simulink model "final"  (R2025b)
settings: Solver=FixedStepAuto  StartTime=0.0  StopTime=20.0  FixedStep=0.001  RelTol=1e-3
values from neighbouring files (symbols this model uses):
  c_d = 0.05    [final_param.m]
  Dm = 1e-3    (= 0.001)    [final_param.m]
  Jm = 0.1e-3    (= 0.0001)    [final_param.m]
  k_s = 0.2    [final_param.m]
  L = [L11]    [final_param.m]
  Ld = 0.01    [final_param.m]
  Lq = 0.02    [final_param.m]
  p = 2    [final_param.m]
  Phi = 0.1    [final_param.m]
  Rs = 0.38    [final_param.m]
libraries: fl_lib x50, nesl_utility x50, ee_lib x15, eeTransforms x10, simulink x1
(part 3 of 3)

== system final/Subsystem5/Plant/MechSensor ==
  Ideal Rotational Motion Sensor : fl_lib/Mechanical/Mechanical Sensors/Ideal Rotational Motion Sensor  reference=foundation.enum.MeasurementReference.difference  acceleration_port=false  velocity_port=true  position_port=true  wrap_angle=simscape.enum.onoff.off  offset=0 rad
  Ideal Torque Sensor : fl_lib/Mechanical/Mechanical Sensors/Ideal Torque Sensor
  PS-Simulink Converter : nesl_utility/PS-Simulink Converter  PhysicalDomain=network_engine_domain  SubClassName=ps_output  LeftPortType=input  RightPortType=output  PseudoPeriodic=off  Frequencies=[]  VectorFormat=1-D array  Unit=1  AffineConversion=off
  PS-Simulink Converter1 : nesl_utility/PS-Simulink Converter  PhysicalDomain=network_engine_domain  SubClassName=ps_output  LeftPortType=input  RightPortType=output  PseudoPeriodic=off  Frequencies=[]  VectorFormat=1-D array  Unit=1  AffineConversion=off
  PS-Simulink Converter2 : nesl_utility/PS-Simulink Converter  PhysicalDomain=network_engine_domain  SubClassName=ps_output  LeftPortType=input  RightPortType=output  PseudoPeriodic=off  Frequencies=[]  VectorFormat=1-D array  Unit=1  AffineConversion=off
  R1 : PMIOPort  Side=Left
  C1 : PMIOPort  Port=2  Side=Left
  R2 : PMIOPort  Port=3  Side=Right
  C2 : PMIOPort  Port=4  Side=Right
  wm : Outport  VectorParamsAs1DForOutWhenUnconnected=off
  thm : Outport  Port=2  VectorParamsAs1DForOutWhenUnconnected=off
  Tm : Outport  Port=3  VectorParamsAs1DForOutWhenUnconnected=off
  wires:
  PS-Simulink Converter/1 -> thm/1
  PS-Simulink Converter1/1 -> Tm/1
  PS-Simulink Converter2/1 -> wm/1
  connections:
  Ideal Rotational Motion Sensor/RConn3 -- PS-Simulink Converter/LConn1
  Ideal Rotational Motion Sensor/RConn1 -- C2/RConn1 -- C1/RConn1
  Ideal Torque Sensor/LConn1 -- R1/RConn1
  Ideal Torque Sensor/RConn1 -- R2/RConn1 -- Ideal Rotational Motion Sensor/LConn1
  PS-Simulink Converter1/LConn1 -- Ideal Torque Sensor/RConn2
  Ideal Rotational Motion Sensor/RConn2 -- PS-Simulink Converter2/LConn1

== system final/Subsystem1/Controller2/DriverPeripherals/Break Algebraic Loop ==
  In1 : Inport
  Demux : Demux  Outputs=3
  Mux : Mux  Inputs=3
  Transfer Fcn : TransferFcn  Denominator=[1e-6 1]
  Transfer Fcn1 : TransferFcn  Denominator=[1e-6 1]
  Transfer Fcn2 : TransferFcn  Denominator=[1e-6 1]
  Out1 : Outport
  wires:
  In1/1 -> Demux/1
  Demux/1 -> Transfer Fcn/1
  Transfer Fcn/1 -> Mux/1
  Demux/2 -> Transfer Fcn1/1
  Transfer Fcn1/1 -> Mux/2
  Demux/3 -> Transfer Fcn2/1
  Transfer Fcn2/1 -> Mux/3
  Mux/1 -> Out1/1

== system final/Subsystem1/Controller2/FOC/CurrentController ==
  Iqref : Inport
  Id : Inport  Port=2
  Iq : Inport  Port=3
  we : Inport  Port=4
  Integrator : Integrator
  MATLAB Function : MATLAB Function  TreatAsAtomicUnit=on
  Scope : Scope
      settings: ActiveDisplayYMinimum=-0.021972241997855933  ActiveDisplayYMaximum=0.011100987286103392  DataLoggingVariableName=ScopeData15
  Vdref : Outport  VectorParamsAs1DForOutWhenUnconnected=off
  Vqref : Outport  Port=2  VectorParamsAs1DForOutWhenUnconnected=off
  wires:
  MATLAB Function/2(Vd) -> Vdref/1
  Iqref/1 -> MATLAB Function/2(i_q_ref)
  MATLAB Function/4(e_q_bar) -> Scope/1
  we/1 -> MATLAB Function/5(we)
  Id/1 -> MATLAB Function/4(i_d)
  Iq/1 -> MATLAB Function/3(i_q)
  Integrator/1 -> MATLAB Function/1(z_q)
  MATLAB Function/1(Vq) -> Vqref/1
  MATLAB Function/3(dz_q) -> Integrator/1

== system final/Subsystem1/Controller2/FOC/VelocityController ==
  wmref : Inport
  wm : Inport  Port=2
  Gain : Gain  Gain=1/(3/2*p*Phi)
  Integrator : Integrator
  Integrator1 : Integrator
  MATLAB Function : MATLAB Function  TreatAsAtomicUnit=on
  Iqref : Outport  VectorParamsAs1DForOutWhenUnconnected=off
  wires:
  MATLAB Function/2(dot_bar_w) -> Integrator/1
  wm/1 -> MATLAB Function/2(w_m)
  MATLAB Function/1(u_cmd) -> Gain/1
  Integrator/1 -> MATLAB Function/3(bar_w)
  Gain/1 -> Iqref/1
  wmref/1 -> MATLAB Function/1(w_ref)
  MATLAB Function/3(dot_xi) -> Integrator1/1
  Integrator1/1 -> MATLAB Function/4(xi)

== system final/Subsystem1/Controller2/FOC/abc2dq ==
  Iabc : Inport
  thetae : Inport  Port=2
  Demux1 : Demux  Outputs=3
  Park Transform : eeTransforms/Park Transform  AxisAlignment=D-axis  PowerInvariant=off
  Terminator : Terminator
  Id : Outport  VectorParamsAs1DForOutWhenUnconnected=off
  Iq : Outport  Port=2  VectorParamsAs1DForOutWhenUnconnected=off
  wires:
  Iabc/1 -> Park Transform/1
  thetae/1 -> Park Transform/2
  Demux1/3 -> Terminator/1
  Park Transform/1 -> Demux1/1
  Demux1/1 -> Id/1
  Demux1/2 -> Iq/1

== system final/Subsystem1/Controller2/FOC/dq2abc ==
  Vd : Inport
  Vq : Inport  Port=2
  thetae : Inport  Port=3
  Constant : Constant  Value=0
  Inverse Park Transform : eeTransforms/Inverse Park Transform  AxisAlignment=D-axis  PowerInvariant=off
  Mux : Mux  Inputs=3
  Vabc : Outport  VectorParamsAs1DForOutWhenUnconnected=off
  wires:
  thetae/1 -> Inverse Park Transform/2
  Constant/1 -> Mux/3
  Mux/1 -> Inverse Park Transform/1
  Vd/1 -> Mux/1
  Inverse Park Transform/1 -> Vabc/1
  Vq/1 -> Mux/2

== system final/Subsystem1/Controller2/FOC/thm2the ==
  thm : Inport
  Constant : Constant  Value=2*pi
  Mod : Math  Operator=mod  SignedPower=on
  PolePairs : Gain  Gain=p
  the : Outport  VectorParamsAs1DForOutWhenUnconnected=off
  wires:
  Constant/1 -> Mod/2
  PolePairs/1 -> Mod/1
  Mod/1 -> the/1
  thm/1 -> PolePairs/1

== system final/Subsystem1/Controller2/FOC/wm2we ==
  wm : Inport
  PolePairs : Gain  Gain=p
  we : Outport  VectorParamsAs1DForOutWhenUnconnected=off
  wires:
  wm/1 -> PolePairs/1
  PolePairs/1 -> we/1

== system final/Subsystem2/Controller2/DriverPeripherals/Break Algebraic Loop ==
  In1 : Inport
  Demux : Demux  Outputs=3
  Mux : Mux  Inputs=3
  Transfer Fcn : TransferFcn  Denominator=[1e-6 1]
  Transfer Fcn1 : TransferFcn  Denominator=[1e-6 1]
  Transfer Fcn2 : TransferFcn  Denominator=[1e-6 1]
  Out1 : Outport
  wires:
  In1/1 -> Demux/1
  Demux/1 -> Transfer Fcn/1
  Transfer Fcn/1 -> Mux/1
  Demux/2 -> Transfer Fcn1/1
  Transfer Fcn1/1 -> Mux/2
  Demux/3 -> Transfer Fcn2/1
  Transfer Fcn2/1 -> Mux/3
  Mux/1 -> Out1/1

== system final/Subsystem2/Controller2/FOC/CurrentController ==
  Iqref : Inport
  Id : Inport  Port=2
  Iq : Inport  Port=3
  we : Inport  Port=4
  Integrator : Integrator
  MATLAB Function : MATLAB Function  TreatAsAtomicUnit=on
  Scope : Scope
      settings: ActiveDisplayYMinimum=-0.021972241997855933  ActiveDisplayYMaximum=0.011100987286103392  DataLoggingVariableName=ScopeData15
  Vdref : Outport  VectorParamsAs1DForOutWhenUnconnected=off
  Vqref : Outport  Port=2  VectorParamsAs1DForOutWhenUnconnected=off
  wires:
  MATLAB Function/2(Vd) -> Vdref/1
  Iqref/1 -> MATLAB Function/2(i_q_ref)
  MATLAB Function/4(e_q_bar) -> Scope/1
  we/1 -> MATLAB Function/5(we)
  Id/1 -> MATLAB Function/4(i_d)
  Iq/1 -> MATLAB Function/3(i_q)
  Integrator/1 -> MATLAB Function/1(z_q)
  MATLAB Function/1(Vq) -> Vqref/1
  MATLAB Function/3(dz_q) -> Integrator/1

== system final/Subsystem2/Controller2/FOC/VelocityController ==
  wmref : Inport
  wm : Inport  Port=2
  Gain : Gain  Gain=1/(3/2*p*Phi)
  Integrator : Integrator
  Integrator1 : Integrator
  MATLAB Function : MATLAB Function  TreatAsAtomicUnit=on
  Iqref : Outport  VectorParamsAs1DForOutWhenUnconnected=off
  wires:
  MATLAB Function/2(dot_bar_w) -> Integrator/1
  wm/1 -> MATLAB Function/2(w_m)
  MATLAB Function/1(u_cmd) -> Gain/1
  Integrator/1 -> MATLAB Function/3(bar_w)
  Gain/1 -> Iqref/1
  wmref/1 -> MATLAB Function/1(w_ref)
  MATLAB Function/3(dot_xi) -> Integrator1/1
  Integrator1/1 -> MATLAB Function/4(xi)

== system final/Subsystem2/Controller2/FOC/abc2dq ==
  Iabc : Inport
  thetae : Inport  Port=2
  Demux1 : Demux  Outputs=3
  Park Transform : eeTransforms/Park Transform  AxisAlignment=D-axis  PowerInvariant=off
  Terminator : Terminator
  Id : Outport  VectorParamsAs1DForOutWhenUnconnected=off
  Iq : Outport  Port=2  VectorParamsAs1DForOutWhenUnconnected=off
  wires:
  Iabc/1 -> Park Transform/1
  thetae/1 -> Park Transform/2
  Demux1/3 -> Terminator/1
  Park Transform/1 -> Demux1/1
  Demux1/1 -> Id/1
  Demux1/2 -> Iq/1

== system final/Subsystem2/Controller2/FOC/dq2abc ==
  Vd : Inport
  Vq : Inport  Port=2
  thetae : Inport  Port=3
  Constant : Constant  Value=0
  Inverse Park Transform : eeTransforms/Inverse Park Transform  AxisAlignment=D-axis  PowerInvariant=off
  Mux : Mux  Inputs=3
  Vabc : Outport  VectorParamsAs1DForOutWhenUnconnected=off
  wires:
  thetae/1 -> Inverse Park Transform/2
  Constant/1 -> Mux/3
  Mux/1 -> Inverse Park Transform/1
  Vd/1 -> Mux/1
  Inverse Park Transform/1 -> Vabc/1
  Vq/1 -> Mux/2

== system final/Subsystem2/Controller2/FOC/thm2the ==
  thm : Inport
  Constant : Constant  Value=2*pi
  Mod : Math  Operator=mod  SignedPower=on
  PolePairs : Gain  Gain=p
  the : Outport  VectorParamsAs1DForOutWhenUnconnected=off
  wires:
  Constant/1 -> Mod/2
  PolePairs/1 -> Mod/1
  Mod/1 -> the/1
  thm/1 -> PolePairs/1

== system final/Subsystem2/Controller2/FOC/wm2we ==
  wm : Inport
  PolePairs : Gain  Gain=p
  we : Outport  VectorParamsAs1DForOutWhenUnconnected=off
  wires:
  wm/1 -> PolePairs/1
  PolePairs/1 -> we/1

== system final/Subsystem3/Controller2/DriverPeripherals/Break Algebraic Loop ==
  In1 : Inport
  Demux : Demux  Outputs=3
  Mux : Mux  Inputs=3
  Transfer Fcn : TransferFcn  Denominator=[1e-6 1]
  Transfer Fcn1 : TransferFcn  Denominator=[1e-6 1]
  Transfer Fcn2 : TransferFcn  Denominator=[1e-6 1]
  Out1 : Outport
  wires:
  In1/1 -> Demux/1
  Demux/1 -> Transfer Fcn/1
  Transfer Fcn/1 -> Mux/1
  Demux/2 -> Transfer Fcn1/1
  Transfer Fcn1/1 -> Mux/2
  Demux/3 -> Transfer Fcn2/1
  Transfer Fcn2/1 -> Mux/3
  Mux/1 -> Out1/1

== system final/Subsystem3/Controller2/FOC/CurrentController ==
  Iqref : Inport
  Id : Inport  Port=2
  Iq : Inport  Port=3
  we : Inport  Port=4
  Integrator : Integrator
  MATLAB Function : MATLAB Function  TreatAsAtomicUnit=on
  Scope : Scope
      settings: ActiveDisplayYMinimum=-0.021972241997855933  ActiveDisplayYMaximum=0.011100987286103392  DataLoggingVariableName=ScopeData15
  Vdref : Outport  VectorParamsAs1DForOutWhenUnconnected=off
  Vqref : Outport  Port=2  VectorParamsAs1DForOutWhenUnconnected=off
  wires:
  MATLAB Function/2(Vd) -> Vdref/1
  Iqref/1 -> MATLAB Function/2(i_q_ref)
  MATLAB Function/4(e_q_bar) -> Scope/1
  we/1 -> MATLAB Function/5(we)
  Id/1 -> MATLAB Function/4(i_d)
  Iq/1 -> MATLAB Function/3(i_q)
  Integrator/1 -> MATLAB Function/1(z_q)
  MATLAB Function/1(Vq) -> Vqref/1
  MATLAB Function/3(dz_q) -> Integrator/1

== system final/Subsystem3/Controller2/FOC/VelocityController ==
  wmref : Inport
  wm : Inport  Port=2
  Gain : Gain  Gain=1/(3/2*p*Phi)
  Integrator : Integrator
  Integrator1 : Integrator
  MATLAB Function : MATLAB Function  TreatAsAtomicUnit=on
  Iqref : Outport  VectorParamsAs1DForOutWhenUnconnected=off
  wires:
  MATLAB Function/2(dot_bar_w) -> Integrator/1
  wm/1 -> MATLAB Function/2(w_m)
  MATLAB Function/1(u_cmd) -> Gain/1
  Integrator/1 -> MATLAB Function/3(bar_w)
  Gain/1 -> Iqref/1
  wmref/1 -> MATLAB Function/1(w_ref)
  MATLAB Function/3(dot_xi) -> Integrator1/1
  Integrator1/1 -> MATLAB Function/4(xi)

== system final/Subsystem3/Controller2/FOC/abc2dq ==
  Iabc : Inport
  thetae : Inport  Port=2
  Demux1 : Demux  Outputs=3
  Park Transform : eeTransforms/Park Transform  AxisAlignment=D-axis  PowerInvariant=off
  Terminator : Terminator
  Id : Outport  VectorParamsAs1DForOutWhenUnconnected=off
  Iq : Outport  Port=2  VectorParamsAs1DForOutWhenUnconnected=off
  wires:
  Iabc/1 -> Park Transform/1
  thetae/1 -> Park Transform/2
  Demux1/3 -> Terminator/1
  Park Transform/1 -> Demux1/1
  Demux1/1 -> Id/1
  Demux1/2 -> Iq/1

== system final/Subsystem3/Controller2/FOC/dq2abc ==
  Vd : Inport
  Vq : Inport  Port=2
  thetae : Inport  Port=3
  Constant : Constant  Value=0
  Inverse Park Transform : eeTransforms/Inverse Park Transform  AxisAlignment=D-axis  PowerInvariant=off
  Mux : Mux  Inputs=3
  Vabc : Outport  VectorParamsAs1DForOutWhenUnconnected=off
  wires:
  thetae/1 -> Inverse Park Transform/2
  Constant/1 -> Mux/3
  Mux/1 -> Inverse Park Transform/1
  Vd/1 -> Mux/1
  Inverse Park Transform/1 -> Vabc/1
  Vq/1 -> Mux/2

== system final/Subsystem3/Controller2/FOC/thm2the ==
  thm : Inport
  Constant : Constant  Value=2*pi
  Mod : Math  Operator=mod  SignedPower=on
  PolePairs : Gain  Gain=p
  the : Outport  VectorParamsAs1DForOutWhenUnconnected=off
  wires:
  Constant/1 -> Mod/2
  PolePairs/1 -> Mod/1
  Mod/1 -> the/1
  thm/1 -> PolePairs/1

== system final/Subsystem3/Controller2/FOC/wm2we ==
  wm : Inport
  PolePairs : Gain  Gain=p
  we : Outport  VectorParamsAs1DForOutWhenUnconnected=off
  wires:
  wm/1 -> PolePairs/1
  PolePairs/1 -> we/1

== system final/Subsystem4/Controller2/DriverPeripherals/Break Algebraic Loop ==
  In1 : Inport
  Demux : Demux  Outputs=3
  Mux : Mux  Inputs=3
  Transfer Fcn : TransferFcn  Denominator=[1e-6 1]
  Transfer Fcn1 : TransferFcn  Denominator=[1e-6 1]
  Transfer Fcn2 : TransferFcn  Denominator=[1e-6 1]
  Out1 : Outport
  wires:
  In1/1 -> Demux/1
  Demux/1 -> Transfer Fcn/1
  Transfer Fcn/1 -> Mux/1
  Demux/2 -> Transfer Fcn1/1
  Transfer Fcn1/1 -> Mux/2
  Demux/3 -> Transfer Fcn2/1
  Transfer Fcn2/1 -> Mux/3
  Mux/1 -> Out1/1

== system final/Subsystem4/Controller2/FOC/CurrentController ==
  Iqref : Inport
  Id : Inport  Port=2
  Iq : Inport  Port=3
  we : Inport  Port=4
  Integrator : Integrator
  MATLAB Function : MATLAB Function  TreatAsAtomicUnit=on
  Scope : Scope
      settings: ActiveDisplayYMinimum=-0.021972241997855933  ActiveDisplayYMaximum=0.011100987286103392  DataLoggingVariableName=ScopeData15
  Vdref : Outport  VectorParamsAs1DForOutWhenUnconnected=off
  Vqref : Outport  Port=2  VectorParamsAs1DForOutWhenUnconnected=off
  wires:
  MATLAB Function/2(Vd) -> Vdref/1
  Iqref/1 -> MATLAB Function/2(i_q_ref)
  MATLAB Function/4(e_q_bar) -> Scope/1
  we/1 -> MATLAB Function/5(we)
  Id/1 -> MATLAB Function/4(i_d)
  Iq/1 -> MATLAB Function/3(i_q)
  Integrator/1 -> MATLAB Function/1(z_q)
  MATLAB Function/1(Vq) -> Vqref/1
  MATLAB Function/3(dz_q) -> Integrator/1

== system final/Subsystem4/Controller2/FOC/VelocityController ==
  wmref : Inport
  wm : Inport  Port=2
  Gain : Gain  Gain=1/(3/2*p*Phi)
  Integrator : Integrator
  Integrator1 : Integrator
  MATLAB Function : MATLAB Function  TreatAsAtomicUnit=on
  Iqref : Outport  VectorParamsAs1DForOutWhenUnconnected=off
  wires:
  MATLAB Function/2(dot_bar_w) -> Integrator/1
  wm/1 -> MATLAB Function/2(w_m)
  MATLAB Function/1(u_cmd) -> Gain/1
  Integrator/1 -> MATLAB Function/3(bar_w)
  Gain/1 -> Iqref/1
  wmref/1 -> MATLAB Function/1(w_ref)
  MATLAB Function/3(dot_xi) -> Integrator1/1
  Integrator1/1 -> MATLAB Function/4(xi)

== system final/Subsystem4/Controller2/FOC/abc2dq ==
  Iabc : Inport
  thetae : Inport  Port=2
  Demux1 : Demux  Outputs=3
  Park Transform : eeTransforms/Park Transform  AxisAlignment=D-axis  PowerInvariant=off
  Terminator : Terminator
  Id : Outport  VectorParamsAs1DForOutWhenUnconnected=off
  Iq : Outport  Port=2  VectorParamsAs1DForOutWhenUnconnected=off
  wires:
  Iabc/1 -> Park Transform/1
  thetae/1 -> Park Transform/2
  Demux1/3 -> Terminator/1
  Park Transform/1 -> Demux1/1
  Demux1/1 -> Id/1
  Demux1/2 -> Iq/1

== system final/Subsystem4/Controller2/FOC/dq2abc ==
  Vd : Inport
  Vq : Inport  Port=2
  thetae : Inport  Port=3
  Constant : Constant  Value=0
  Inverse Park Transform : eeTransforms/Inverse Park Transform  AxisAlignment=D-axis  PowerInvariant=off
  Mux : Mux  Inputs=3
  Vabc : Outport  VectorParamsAs1DForOutWhenUnconnected=off
  wires:
  thetae/1 -> Inverse Park Transform/2
  Constant/1 -> Mux/3
  Mux/1 -> Inverse Park Transform/1
  Vd/1 -> Mux/1
  Inverse Park Transform/1 -> Vabc/1
  Vq/1 -> Mux/2

== system final/Subsystem4/Controller2/FOC/thm2the ==
  thm : Inport
  Constant : Constant  Value=2*pi
  Mod : Math  Operator=mod  SignedPower=on
  PolePairs : Gain  Gain=p
  the : Outport  VectorParamsAs1DForOutWhenUnconnected=off
  wires:
  Constant/1 -> Mod/2
  PolePairs/1 -> Mod/1
  Mod/1 -> the/1
  thm/1 -> PolePairs/1

== system final/Subsystem4/Controller2/FOC/wm2we ==
  wm : Inport
  PolePairs : Gain  Gain=p
  we : Outport  VectorParamsAs1DForOutWhenUnconnected=off
  wires:
  wm/1 -> PolePairs/1
  PolePairs/1 -> we/1

== system final/Subsystem5/Controller2/DriverPeripherals/Break Algebraic Loop ==
  In1 : Inport
  Demux : Demux  Outputs=3
  Mux : Mux  Inputs=3
  Transfer Fcn : TransferFcn  Denominator=[1e-6 1]
  Transfer Fcn1 : TransferFcn  Denominator=[1e-6 1]
  Transfer Fcn2 : TransferFcn  Denominator=[1e-6 1]
  Out1 : Outport
  wires:
  In1/1 -> Demux/1
  Demux/1 -> Transfer Fcn/1
  Transfer Fcn/1 -> Mux/1
  Demux/2 -> Transfer Fcn1/1
  Transfer Fcn1/1 -> Mux/2
  Demux/3 -> Transfer Fcn2/1
  Transfer Fcn2/1 -> Mux/3
  Mux/1 -> Out1/1

== system final/Subsystem5/Controller2/FOC/CurrentController ==
  Iqref : Inport
  Id : Inport  Port=2
  Iq : Inport  Port=3
  we : Inport  Port=4
  Integrator : Integrator
  MATLAB Function : MATLAB Function  TreatAsAtomicUnit=on
  Scope : Scope
      settings: ActiveDisplayYMinimum=-0.021972241997855933  ActiveDisplayYMaximum=0.011100987286103392  DataLoggingVariableName=ScopeData15
  Vdref : Outport  VectorParamsAs1DForOutWhenUnconnected=off
  Vqref : Outport  Port=2  VectorParamsAs1DForOutWhenUnconnected=off
  wires:
  MATLAB Function/2(Vd) -> Vdref/1
  Iqref/1 -> MATLAB Function/2(i_q_ref)
  MATLAB Function/4(e_q_bar) -> Scope/1
  we/1 -> MATLAB Function/5(we)
  Id/1 -> MATLAB Function/4(i_d)
  Iq/1 -> MATLAB Function/3(i_q)
  Integrator/1 -> MATLAB Function/1(z_q)
  MATLAB Function/1(Vq) -> Vqref/1
  MATLAB Function/3(dz_q) -> Integrator/1

== system final/Subsystem5/Controller2/FOC/VelocityController ==
  wmref : Inport
  wm : Inport  Port=2
  Gain : Gain  Gain=1/(3/2*p*Phi)
  Integrator : Integrator
  Integrator1 : Integrator
  MATLAB Function : MATLAB Function  TreatAsAtomicUnit=on
  Iqref : Outport  VectorParamsAs1DForOutWhenUnconnected=off
  wires:
  MATLAB Function/2(dot_bar_w) -> Integrator/1
  wm/1 -> MATLAB Function/2(w_m)
  MATLAB Function/1(u_cmd) -> Gain/1
  Integrator/1 -> MATLAB Function/3(bar_w)
  Gain/1 -> Iqref/1
  wmref/1 -> MATLAB Function/1(w_ref)
  MATLAB Function/3(dot_xi) -> Integrator1/1
  Integrator1/1 -> MATLAB Function/4(xi)

== system final/Subsystem5/Controller2/FOC/abc2dq ==
  Iabc : Inport
  thetae : Inport  Port=2
  Demux1 : Demux  Outputs=3
  Park Transform : eeTransforms/Park Transform  AxisAlignment=D-axis  PowerInvariant=off
  Terminator : Terminator
  Id : Outport  VectorParamsAs1DForOutWhenUnconnected=off
  Iq : Outport  Port=2  VectorParamsAs1DForOutWhenUnconnected=off
  wires:
  Iabc/1 -> Park Transform/1
  thetae/1 -> Park Transform/2
  Demux1/3 -> Terminator/1
  Park Transform/1 -> Demux1/1
  Demux1/1 -> Id/1
  Demux1/2 -> Iq/1

== system final/Subsystem5/Controller2/FOC/dq2abc ==
  Vd : Inport
  Vq : Inport  Port=2
  thetae : Inport  Port=3
  Constant : Constant  Value=0
  Inverse Park Transform : eeTransforms/Inverse Park Transform  AxisAlignment=D-axis  PowerInvariant=off
  Mux : Mux  Inputs=3
  Vabc : Outport  VectorParamsAs1DForOutWhenUnconnected=off
  wires:
  thetae/1 -> Inverse Park Transform/2
  Constant/1 -> Mux/3
  Mux/1 -> Inverse Park Transform/1
  Vd/1 -> Mux/1
  Inverse Park Transform/1 -> Vabc/1
  Vq/1 -> Mux/2

== system final/Subsystem5/Controller2/FOC/thm2the ==
  thm : Inport
  Constant : Constant  Value=2*pi
  Mod : Math  Operator=mod  SignedPower=on
  PolePairs : Gain  Gain=p
  the : Outport  VectorParamsAs1DForOutWhenUnconnected=off
  wires:
  Constant/1 -> Mod/2
  PolePairs/1 -> Mod/1
  Mod/1 -> the/1
  thm/1 -> PolePairs/1

== system final/Subsystem5/Controller2/FOC/wm2we ==
  wm : Inport
  PolePairs : Gain  Gain=p
  we : Outport  VectorParamsAs1DForOutWhenUnconnected=off
  wires:
  wm/1 -> PolePairs/1
  PolePairs/1 -> we/1

== matlab function final/Subsystem4/Controller2/FOC/CurrentController/MATLAB Function ==
  data: z_q input; Vq output; i_q_ref input; i_q input; i_d input; we input; Vd output; dz_q output; e_q_bar output; Rs parameter; Ld parameter; Lq parameter; Phi parameter
function [Vq, Vd, dz_q, e_q_bar] = smc_ctrl(z_q, i_q_ref, i_q, i_d, we, Rs, Ld, Lq, Phi)
%#codegen
% ============================================================
%  PMSM 超螺旋滑模电流控制器
%  Rs, Ld, Lq, Phi, p 及滑模增益均由 Parameter 作用域提供
% ============================================================

%% ---------- 滑模参数 (仍然写死, 因为它们只属于控制器) ----------
r1  = 0.5;   r2  = 1.5;
rho1 = 0.5;  rho2 = 1.5;

k_q1 = -5000;  k_q2 = -4000;
k_d1 = -5000;  k_d2 = -4000;

lam_q1 = 50;   lam_q2 = 50;

%% ---------- 滑模面 ----------
e_q_bar = i_q - z_q;

%% ---------- 迭代部分的导数 (积分交给 Simulink) ----------
e_z  = z_q - i_q_ref;
dz_q = -lam_q1 * sig(e_z, rho1) - lam_q2 * sig(e_z, rho2);

%% ---------- u_q (非迭代) ----------
Vq = Lq * ( dz_q ...
             + k_q1 * sig(e_q_bar, r1) ...
             + k_q2 * sig(e_q_bar, r2) ) ...
      + Rs * z_q ...
      + Ld * we * i_d ...
      + we * Phi ;

%% ---------- u_d (非迭代) ----------
Vd = Ld * ( k_d1 * sig(i_d, r1) ...
             + k_d2 * sig(i_d, r2) ) ...
      + Rs * i_d ...
      + Lq * we * i_q;

end

function y = sig(x, r)
    y = abs(x)^r * sign(x);
end

== matlab function final/Subsystem4/Controller2/FOC/VelocityController/MATLAB Function ==
  data: w_ref input; u_cmd output; w_m input; bar_w input; xi input; Jm parameter; Dm parameter; dot_bar_w output; dot_xi output
function [u_cmd, dot_bar_w, dot_xi] = FixedTimeController(w_ref, w_m, bar_w, xi, Jm, Dm)

    lambda1  = 5;   lambda2 = 5;   lambda3 = 6;
    tau      = 0.5; vartheta = 1.5;
    k_w = 6; k1 = 5; k2 = 5;

    k_i = 20;

    kappa0 = 30;     % 线性积分增益（新增，压制小误差）
    kappa1 = 20;     % 固定时间项增益
    kappa2 = 20;
    alpha1 = 0.5;
    alpha2 = 1.5;

    pow_func = @(x, gamma) abs(x)^gamma * sign(x);

    % 公式(117) 滤波器
    e_w = bar_w - w_ref;
    dot_bar_w = (1/tau) * ( -lambda1 * pow_func(e_w, 0.5) ...
                            -lambda2 * pow_func(e_w, vartheta) ...
                            -lambda3 * e_w );

    s   = w_m - bar_w;
    e_v = w_m - w_ref;

    % 混合固定时间积分
    dot_xi = kappa0 * e_v ...
           + kappa1 * pow_func(e_v, alpha1) ...
           + kappa2 * pow_func(e_v, alpha2);

    TL_hat_int = k_i * xi;

    feedback = -k_w * s ...
               - k1 * pow_func(s, 0.5) ...
               - k2 * pow_func(s, vartheta);

    u_cmd = Jm * dot_bar_w + Dm * bar_w - TL_hat_int + feedback;
end

== matlab function final/Subsystem2/Controller2/FOC/CurrentController/MATLAB Function ==
  data: z_q input; Vq output; i_q_ref input; i_q input; i_d input; we input; Vd output; dz_q output; e_q_bar output; Rs parameter; Ld parameter; Lq parameter; Phi parameter
function [Vq, Vd, dz_q, e_q_bar] = smc_ctrl(z_q, i_q_ref, i_q, i_d, we, Rs, Ld, Lq, Phi)
%#codegen
% ============================================================
%  PMSM 超螺旋滑模电流控制器
%  Rs, Ld, Lq, Phi, p 及滑模增益均由 Parameter 作用域提供
% ============================================================

%% ---------- 滑模参数 (仍然写死, 因为它们只属于控制器) ----------
r1  = 0.5;   r2  = 1.5;
rho1 = 0.5;  rho2 = 1.5;

k_q1 = -5000;  k_q2 = -4000;
k_d1 = -5000;  k_d2 = -4000;

lam_q1 = 50;   lam_q2 = 50;

%% ---------- 滑模面 ----------
e_q_bar = i_q - z_q;

%% ---------- 迭代部分的导数 (积分交给 Simulink) ----------
e_z  = z_q - i_q_ref;
dz_q = -lam_q1 * sig(e_z, rho1) - lam_q2 * sig(e_z, rho2);

%% ---------- u_q (非迭代) ----------
Vq = Lq * ( dz_q ...
             + k_q1 * sig(e_q_bar, r1) ...
             + k_q2 * sig(e_q_bar, r2) ) ...
      + Rs * z_q ...
      + Ld * we * i_d ...
      + we * Phi ;

%% ---------- u_d (非迭代) ----------
Vd = Ld * ( k_d1 * sig(i_d, r1) ...
             + k_d2 * sig(i_d, r2) ) ...
      + Rs * i_d ...
      + Lq * we * i_q;

end

function y = sig(x, r)
    y = abs(x)^r * sign(x);
end

== matlab function final/Subsystem/MATLAB Function ==
  data: theta input; w input; couple output; L parameter; k_s parameter; c_d parameter
function couple = couple(theta,w, L, k_s, c_d)

couple = -L * (k_s*theta +  c_d * w);

== matlab function final/Subsystem2/Controller2/FOC/VelocityController/MATLAB Function ==
  data: w_ref input; u_cmd output; w_m input; bar_w input; xi input; Jm parameter; Dm parameter; dot_bar_w output; dot_xi output
function [u_cmd, dot_bar_w, dot_xi] = FixedTimeController(w_ref, w_m, bar_w, xi, Jm, Dm)

    lambda1  = 5;   lambda2 = 5;   lambda3 = 6;
    tau      = 0.5; vartheta = 1.5;
    k_w = 6; k1 = 5; k2 = 5;

    k_i = 20;

    kappa0 = 30;     % 线性积分增益（新增，压制小误差）
    kappa1 = 20;     % 固定时间项增益
    kappa2 = 20;
    alpha1 = 0.5;
    alpha2 = 1.5;

    pow_func = @(x, gamma) abs(x)^gamma * sign(x);

    % 公式(117) 滤波器
    e_w = bar_w - w_ref;
    dot_bar_w = (1/tau) * ( -lambda1 * pow_func(e_w, 0.5) ...
                            -lambda2 * pow_func(e_w, vartheta) ...
                            -lambda3 * e_w );

    s   = w_m - bar_w;
    e_v = w_m - w_ref;

    % 混合固定时间积分
    dot_xi = kappa0 * e_v ...
           + kappa1 * pow_func(e_v, alpha1) ...
           + kappa2 * pow_func(e_v, alpha2);

    TL_hat_int = k_i * xi;

    feedback = -k_w * s ...
               - k1 * pow_func(s, 0.5) ...
               - k2 * pow_func(s, vartheta);

    u_cmd = Jm * dot_bar_w + Dm * bar_w - TL_hat_int + feedback;
end

== matlab function final/Subsystem3/Controller2/FOC/CurrentController/MATLAB Function ==
  data: z_q input; Vq output; i_q_ref input; i_q input; i_d input; we input; Vd output; dz_q output; e_q_bar output; Rs parameter; Ld parameter; Lq parameter; Phi parameter
function [Vq, Vd, dz_q, e_q_bar] = smc_ctrl(z_q, i_q_ref, i_q, i_d, we, Rs, Ld, Lq, Phi)
%#codegen
% ============================================================
%  PMSM 超螺旋滑模电流控制器
%  Rs, Ld, Lq, Phi, p 及滑模增益均由 Parameter 作用域提供
% ============================================================

%% ---------- 滑模参数 (仍然写死, 因为它们只属于控制器) ----------
r1  = 0.5;   r2  = 1.5;
rho1 = 0.5;  rho2 = 1.5;

k_q1 = -5000;  k_q2 = -4000;
k_d1 = -5000;  k_d2 = -4000;

lam_q1 = 50;   lam_q2 = 50;

%% ---------- 滑模面 ----------
e_q_bar = i_q - z_q;

%% ---------- 迭代部分的导数 (积分交给 Simulink) ----------
e_z  = z_q - i_q_ref;
dz_q = -lam_q1 * sig(e_z, rho1) - lam_q2 * sig(e_z, rho2);

%% ---------- u_q (非迭代) ----------
Vq = Lq * ( dz_q ...
             + k_q1 * sig(e_q_bar, r1) ...
             + k_q2 * sig(e_q_bar, r2) ) ...
      + Rs * z_q ...
      + Ld * we * i_d ...
      + we * Phi ;

%% ---------- u_d (非迭代) ----------
Vd = Ld * ( k_d1 * sig(i_d, r1) ...
             + k_d2 * sig(i_d, r2) ) ...
      + Rs * i_d ...
      + Lq * we * i_q;

end

function y = sig(x, r)
    y = abs(x)^r * sign(x);
end

== matlab function final/Subsystem1/Controller2/FOC/CurrentController/MATLAB Function ==
  data: z_q input; Vq output; i_q_ref input; i_q input; i_d input; we input; Vd output; dz_q output; e_q_bar output; Rs parameter; Ld parameter; Lq parameter; Phi parameter
function [Vq, Vd, dz_q, e_q_bar] = smc_ctrl(z_q, i_q_ref, i_q, i_d, we, Rs, Ld, Lq, Phi)
%#codegen
% ============================================================
%  PMSM 超螺旋滑模电流控制器
%  Rs, Ld, Lq, Phi, p 及滑模增益均由 Parameter 作用域提供
% ============================================================

%% ---------- 滑模参数 (仍然写死, 因为它们只属于控制器) ----------
r1  = 0.5;   r2  = 1.5;
rho1 = 0.5;  rho2 = 1.5;

k_q1 = -5000;  k_q2 = -4000;
k_d1 = -5000;  k_d2 = -4000;

lam_q1 = 50;   lam_q2 = 50;

%% ---------- 滑模面 ----------
e_q_bar = i_q - z_q;

%% ---------- 迭代部分的导数 (积分交给 Simulink) ----------
e_z  = z_q - i_q_ref;
dz_q = -lam_q1 * sig(e_z, rho1) - lam_q2 * sig(e_z, rho2);

%% ---------- u_q (非迭代) ----------
Vq = Lq * ( dz_q ...
             + k_q1 * sig(e_q_bar, r1) ...
             + k_q2 * sig(e_q_bar, r2) ) ...
      + Rs * z_q ...
      + Ld * we * i_d ...
      + we * Phi ;

%% ---------- u_d (非迭代) ----------
Vd = Ld * ( k_d1 * sig(i_d, r1) ...
             + k_d2 * sig(i_d, r2) ) ...
      + Rs * i_d ...
      + Lq * we * i_q;

end

function y = sig(x, r)
    y = abs(x)^r * sign(x);
end

== matlab function final/Subsystem3/Controller2/FOC/VelocityController/MATLAB Function ==
  data: w_ref input; u_cmd output; w_m input; bar_w input; xi input; Jm parameter; Dm parameter; dot_bar_w output; dot_xi output
function [u_cmd, dot_bar_w, dot_xi] = FixedTimeController(w_ref, w_m, bar_w, xi, Jm, Dm)

    lambda1  = 5;   lambda2 = 5;   lambda3 = 6;
    tau      = 0.5; vartheta = 1.5;
    k_w = 6; k1 = 5; k2 = 5;

    k_i = 20;

    kappa0 = 30;     % 线性积分增益（新增，压制小误差）
    kappa1 = 20;     % 固定时间项增益
    kappa2 = 20;
    alpha1 = 0.5;
    alpha2 = 1.5;

    pow_func = @(x, gamma) abs(x)^gamma * sign(x);

    % 公式(117) 滤波器
    e_w = bar_w - w_ref;
    dot_bar_w = (1/tau) * ( -lambda1 * pow_func(e_w, 0.5) ...
                            -lambda2 * pow_func(e_w, vartheta) ...
                            -lambda3 * e_w );

    s   = w_m - bar_w;
    e_v = w_m - w_ref;

    % 混合固定时间积分
    dot_xi = kappa0 * e_v ...
           + kappa1 * pow_func(e_v, alpha1) ...
           + kappa2 * pow_func(e_v, alpha2);

    TL_hat_int = k_i * xi;

    feedback = -k_w * s ...
               - k1 * pow_func(s, 0.5) ...
               - k2 * pow_func(s, vartheta);

    u_cmd = Jm * dot_bar_w + Dm * bar_w - TL_hat_int + feedback;
end

== matlab function final/Subsystem5/Controller2/FOC/VelocityController/MATLAB Function ==
  data: w_ref input; u_cmd output; w_m input; bar_w input; xi input; Jm parameter; Dm parameter; dot_bar_w output; dot_xi output
function [u_cmd, dot_bar_w, dot_xi] = FixedTimeController(w_ref, w_m, bar_w, xi, Jm, Dm)

    lambda1  = 5;   lambda2 = 5;   lambda3 = 6;
    tau      = 0.5; vartheta = 1.5;
    k_w = 6; k1 = 5; k2 = 5;

    k_i = 20;

    kappa0 = 30;     % 线性积分增益（新增，压制小误差）
    kappa1 = 20;     % 固定时间项增益
    kappa2 = 20;
    alpha1 = 0.5;
    alpha2 = 1.5;

    pow_func = @(x, gamma) abs(x)^gamma * sign(x);

    % 公式(117) 滤波器
    e_w = bar_w - w_ref;
    dot_bar_w = (1/tau) * ( -lambda1 * pow_func(e_w, 0.5) ...
                            -lambda2 * pow_func(e_w, vartheta) ...
                            -lambda3 * e_w );

    s   = w_m - bar_w;
    e_v = w_m - w_ref;

    % 混合固定时间积分
    dot_xi = kappa0 * e_v ...
           + kappa1 * pow_func(e_v, alpha1) ...
           + kappa2 * pow_func(e_v, alpha2);

    TL_hat_int = k_i * xi;

    feedback = -k_w * s ...
               - k1 * pow_func(s, 0.5) ...
               - k2 * pow_func(s, vartheta);

    u_cmd = Jm * dot_bar_w + Dm * bar_w - TL_hat_int + feedback;
end

== matlab function final/Subsystem6/MATLAB Function3 ==
  data: etheta input; u_t input; u output; u_s input
function u = fcn(etheta, u_t,u_s)
c=0;
u=u_t.*ones(size(u_s))-c*etheta+u_s;

== matlab function final/Subsystem6/MATLAB Function ==
  data: y1 input; y1_dot output; y2 input; y2_dot output
function [y1_dot, y2_dot] = calc_threshold_derivs(y1, y2)
    % 参数定义
    pi1 = 0.6; pi2 = 0.6;
    alpha1 = 0.5; alpha2 = 0.5;
    beta1 = 0.7; beta2 = 0.72;
    mu = 1.55;

    % 确保y1和y2非负（关键修改）
    y1 = max(y1, 0);
    y2 = max(y2, 0);

    % 修正后的独立更新公式
    y1_dot = -pi1*y1 - alpha1*(y1^0.5) - beta1*(y1^((1+mu)/2))+0.01;
    y2_dot = -pi2*y2 - alpha2*(y2^0.5) - beta2*(y2^((1+mu)/2))+0.05;
end

== matlab function final/Subsystem6/MATLAB Function1 ==
  data: theta_vec input; V output
function V = calc_error_energy(theta_vec)
% 输入: 

% 输出: V (标量，复合误差能量)

% 计算跟随者平均角速度
theta_mean = mean(theta_vec);


% 计算同步误差（跟随者间）
phi_sync = theta_vec - theta_mean;

V = sum(phi_sync.^2);
end

== matlab function final/Subsystem6/MATLAB Function2 ==
  settings: updateMethod=DISCRETE  sampleTime=0.001
  data: theta_vec input; u_sync output; V input; Y1 input; Y2 input; L parameter
function u_sync = control_law(theta_vec, V, Y1, Y2, L)
% 输入: 
%   omega_vec (5x1向量，跟随者角速度)
%   V (标量，复合误差能量)
%   Y1, Y2 (标量，动态阈值)
%   omega_leader (标量，领导者角速度)
% 输出: u_out (5x1向量，控制量)

% 强制输入信号为实数
theta_vec = real(theta_vec);

% 参数定义（对应公式2中的β1,β2,β3,θ,δ^k）
beta1 = 10;    % 对应公式中的β1
beta2 = 10;    % 对应公式中的β2
beta3 = 0.0;  % 对应公式中的β3
theta = 1.55; % 对应公式中的θ
delta_k = 0.5;% 对应公式中的δ^k（可调）

% 持久变量（存储状态、初始角速度）
persistent tk sk prev_V prev_Y1 prev_Y2

% 初始化
if isempty(tk)
    tk = 0; sk = 0;
    prev_V = 0; prev_Y1 = 50.0; prev_Y2 = 20.0;
end

% 事件触发逻辑
is_firing = false;
if V >= Y1
    is_firing = true;
    if prev_V < prev_Y1
        tk = tk + 1;
    end
elseif V <= Y2
    is_firing = false;
    if (prev_V > prev_Y2) && (tk > sk)
        sk = sk + 1;
    end
else
    if tk > sk
        is_firing = true;
    else
        is_firing = false;
    end
end

% 更新状态
prev_V = V;
prev_Y1 = Y1;
prev_Y2 = Y2;




n = 5;   % 跟随者数量

if is_firing
    % 状态向量 omega_vec 为 10x1
    % 构造差值矩阵 Diff(i,j) = x_i - x_j
    X_i = repmat(theta_vec, 1, n);          % 10x10
    X_j = repmat(theta_vec.', n, 1);        % 10x10
    Diff = X_i - X_j;                       % 10x10

    % 权重矩阵：直接使用拉普拉斯矩阵 L
    W = -L;

    % 对角线置零，排除自身交互
    W(1:n+1:end) = 0;

    % 第一项：-β1 * δ^k * ∑ W(i,j) * sign(x_i - x_j)
    sum1 = -beta1 * delta_k * sum(W .* sign(Diff), 2);

    % 第二项：-β2 * δ^k * ∑ W(i,j) * sign(x_i - x_j) .* |x_i - x_j|^θ
    sum2 = -beta2 * delta_k * sum(W .* sign(Diff) .* abs(Diff).^theta, 2);

    % 第三项：-β3 * δ^k * ∑ W(i,j) * (x_i - x_j)
    sum3 = -beta3 * delta_k * sum(W .* Diff, 2);

    % 合成控制量
    u_formula2 = sum1 + sum2 + sum3;   % 10x1

    u_sync = u_formula2;
else
    u_sync = zeros(n, 1);
end

end

== matlab function final/Subsystem5/Controller2/FOC/CurrentController/MATLAB Function ==
  data: z_q input; Vq output; i_q_ref input; i_q input; i_d input; we input; Vd output; dz_q output; e_q_bar output; Rs parameter; Ld parameter; Lq parameter; Phi parameter
function [Vq, Vd, dz_q, e_q_bar] = smc_ctrl(z_q, i_q_ref, i_q, i_d, we, Rs, Ld, Lq, Phi)
%#codegen
% ============================================================
%  PMSM 超螺旋滑模电流控制器
%  Rs, Ld, Lq, Phi, p 及滑模增益均由 Parameter 作用域提供
% ============================================================

%% ---------- 滑模参数 (仍然写死, 因为它们只属于控制器) ----------
r1  = 0.5;   r2  = 1.5;
rho1 = 0.5;  rho2 = 1.5;

k_q1 = -5000;  k_q2 = -4000;
k_d1 = -5000;  k_d2 = -4000;

lam_q1 = 50;   lam_q2 = 50;

%% ---------- 滑模面 ----------
e_q_bar = i_q - z_q;

%% ---------- 迭代部分的导数 (积分交给 Simulink) ----------
e_z  = z_q - i_q_ref;
dz_q = -lam_q1 * sig(e_z, rho1) - lam_q2 * sig(e_z, rho2);

%% ---------- u_q (非迭代) ----------
Vq = Lq * ( dz_q ...
             + k_q1 * sig(e_q_bar, r1) ...
             + k_q2 * sig(e_q_bar, r2) ) ...
      + Rs * z_q ...
      + Ld * we * i_d ...
      + we * Phi ;

%% ---------- u_d (非迭代) ----------
Vd = Ld * ( k_d1 * sig(i_d, r1) ...
             + k_d2 * sig(i_d, r2) ) ...
      + Rs * i_d ...
      + Lq * we * i_q;

end

function y = sig(x, r)
    y = abs(x)^r * sign(x);
end

== matlab function final/Subsystem1/Controller2/FOC/VelocityController/MATLAB Function ==
  data: w_ref input; u_cmd output; w_m input; bar_w input; xi input; Jm parameter; Dm parameter; dot_bar_w output; dot_xi output
function [u_cmd, dot_bar_w, dot_xi] = FixedTimeController(w_ref, w_m, bar_w, xi, Jm, Dm)

    lambda1  = 5;   lambda2 = 5;   lambda3 = 6;
    tau      = 0.5; vartheta = 1.5;
    k_w = 6; k1 = 5; k2 = 5;

    k_i = 20;

    kappa0 = 30;     % 线性积分增益（新增，压制小误差）
    kappa1 = 20;     % 固定时间项增益
    kappa2 = 20;
    alpha1 = 0.5;
    alpha2 = 1.5;

    pow_func = @(x, gamma) abs(x)^gamma * sign(x);

    % 公式(117) 滤波器
    e_w = bar_w - w_ref;
    dot_bar_w = (1/tau) * ( -lambda1 * pow_func(e_w, 0.5) ...
                            -lambda2 * pow_func(e_w, vartheta) ...
                            -lambda3 * e_w );

    s   = w_m - bar_w;
    e_v = w_m - w_ref;

    % 混合固定时间积分
    dot_xi = kappa0 * e_v ...
           + kappa1 * pow_func(e_v, alpha1) ...
           + kappa2 * pow_func(e_v, alpha2);

    TL_hat_int = k_i * xi;

    feedback = -k_w * s ...
               - k1 * pow_func(s, 0.5) ...
               - k2 * pow_func(s, vartheta);

    u_cmd = Jm * dot_bar_w + Dm * bar_w - TL_hat_int + feedback;
end
